simulink model "fadingbuttons"  (R2016a)
settings: Solver=FixedStepAuto  StartTime=0.0  StopTime=Inf  RelTol=1e-3
undefined symbols (not defined in the file): DiscIntNeverNeededParam
libraries: arduinolib x2
settings Model: SimulationMode=external  ExtModeTrigDuration=2  Creator=bai  LastModifiedBy=bai
settings OptimizationCC: OptimizeModelRefInitCode=on  LifeSpan=1  MaxStackSize=64
settings HardwareCC: ProdBitPerInt=16  ProdBitPerPointer=16  ProdLargestAtomicFloat=None  ProdWordSize=8  ProdHWDeviceType=Atmel->AVR
settings RTWCC: SystemTargetFile=ert.tlc  HardwareBoard=Arduino Mega 2560  TemplateMakefile=ert_default_tmf  GenerateReport=on  Toolchain=Arduino AVR v1.6.1  BuildConfiguration=Faster Runs  IncludeHyperlinkInReport=on  LaunchReport=on  GenerateTraceInfo=on  GenerateTraceReport=on  GenerateTraceReportSl=on  GenerateTraceReportSf=on  GenerateTraceReportEml=on
settings CodeAppCC: ForceParamTrailComments=on  IgnoreCustomStorageClasses=off  OperatorAnnotations=on  SimulinkDataObjDesc=on  SFDataObjDesc=on  MATLABFcnDesc=on  InsertBlockDesc=on  MATLABSourceComments=on
settings ERTTargetCC: SupportContinuousTime=on  SupportVariableSizeSignals=on

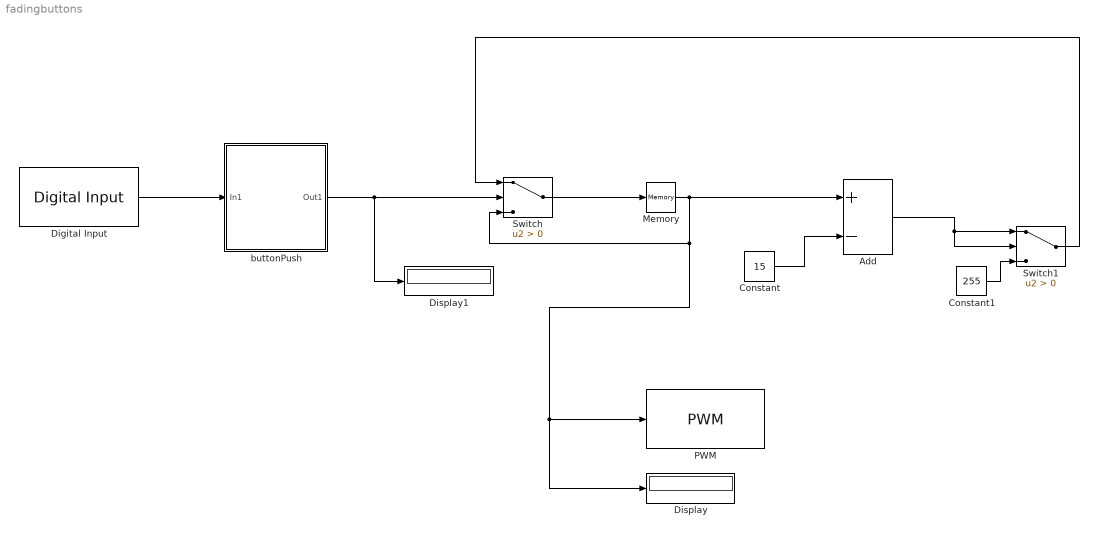
== system fadingbuttons ==
  Add : Sum  Inputs=+-
  Constant : Constant  Value=15  SampleTime=0.01
  Constant1 : Constant  Value=255  SampleTime=0.01
  Digital Input : arduinolib/Digital Input  pinNumber=3  sampleTime=0.01  blockPlatform=arduino
  Display : Display
  Display1 : Display
  Memory : Memory  X0=255
  PWM : arduinolib/PWM  pinNumber=9  blockPlatform=arduino
  Switch : Switch  Criteria=u2 > Threshold
  Switch1 : Switch  Criteria=u2 > Threshold
  "buttonPush " : Subsystem
  wires:
  Digital Input/1 -> "buttonPush "/1(In1)
  "buttonPush "/1(Out1) -> Display1/1, Switch/2
  Switch/1 -> Memory/1
  Memory/1 -> Add/1, Display/1, PWM/1, Switch/3
  Constant/1 -> Add/2
  Constant1/1 -> Switch1/3
  Add/1 -> Switch1/1, Switch1/2
  Switch1/1 -> Switch/1

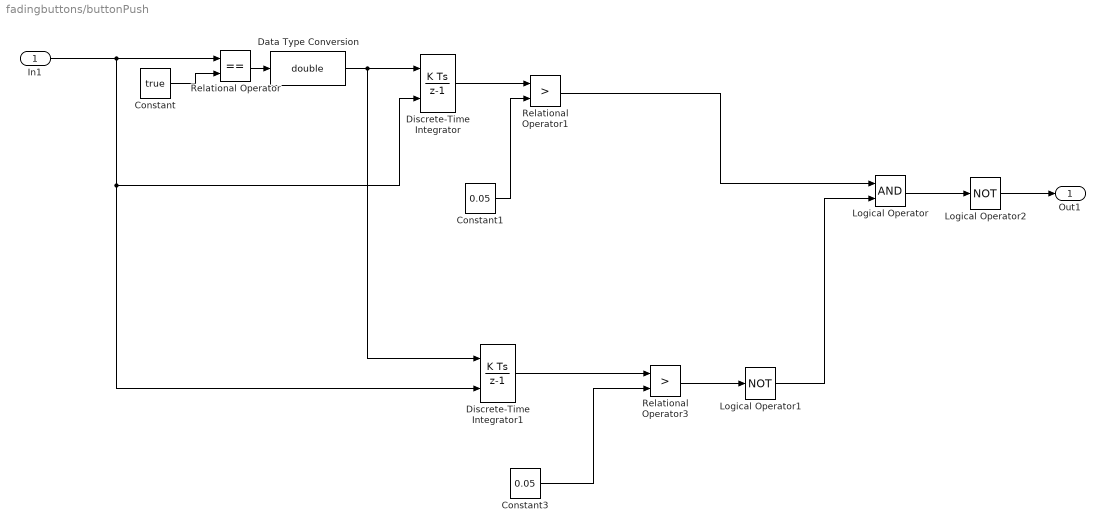
== system fadingbuttons/buttonPush  ==
  In1 : Inport
  Constant : Constant  Value=true  SampleTime=0.01
  Constant1 : Constant  Value=0.05  SampleTime=0.01
  Constant3 : Constant  Value=0.05  SampleTime=0.01
  Data Type Conversion : DataTypeConversion  OutDataTypeStr=double
  Discrete-Time Integrator : DiscreteIntegrator  ExternalReset=rising  InitialConditionSetting=State (most efficient)  SampleTime=0.01  ICPrevOutput=DiscIntNeverNeededParam  ICPrevScaledInput=DiscIntNeverNeededParam
  Discrete-Time Integrator1 : DiscreteIntegrator  ExternalReset=falling  InitialConditionSetting=State (most efficient)  SampleTime=0.01  ICPrevOutput=DiscIntNeverNeededParam  ICPrevScaledInput=DiscIntNeverNeededParam
  Logical Operator : Logic  AllPortsSameDT=off  OutDataTypeStr=boolean
  Logical Operator1 : Logic  Operator=NOT  AllPortsSameDT=off  OutDataTypeStr=boolean
  Logical Operator2 : Logic  Operator=NOT  AllPortsSameDT=off  OutDataTypeStr=boolean
  Relational Operator : RelationalOperator  Operator===  OutDataTypeStr=boolean
  Relational Operator1 : RelationalOperator  Operator=>  OutDataTypeStr=boolean
  Relational Operator3 : RelationalOperator  Operator=>  OutDataTypeStr=boolean
  Out1 : Outport
  wires:
  Discrete-Time Integrator/1 -> Relational Operator1/1
  Constant1/1 -> Relational Operator1/2
  Data Type Conversion/1 -> Discrete-Time Integrator1/1, Discrete-Time Integrator/1
  Constant/1 -> Relational Operator/2
  Relational Operator/1 -> Data Type Conversion/1
  In1/1 -> Discrete-Time Integrator1/2, Discrete-Time Integrator/2, Relational Operator/1
  Constant3/1 -> Relational Operator3/2
  Discrete-Time Integrator1/1 -> Relational Operator3/1
  Relational Operator3/1 -> Logical Operator1/1
  Logical Operator1/1 -> Logical Operator/2
  Relational Operator1/1 -> Logical Operator/1
  Logical Operator/1 -> Logical Operator2/1
  Logical Operator2/1 -> Out1/1
